simulink model "example_of_convert_unit"  (R2021a)
settings: Solver=VariableStepAuto  StartTime=0.0  StopTime=10.0  RelTol=1e-3
settings Model: Creator=YasserNet  LastModifiedBy=YasserNet

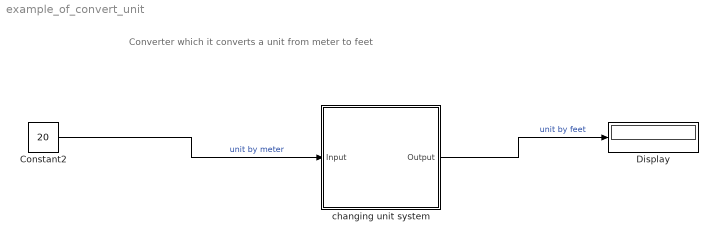
== system example_of_convert_unit ==
  note: Converter which it converts a unit from meter to feet
  Constant2 : Constant  Value=20
  Display : Display
  "changing unit system " : Subsystem
  wires:
  "changing unit system "/1(Output) -> Display/1  "unit by feet"
  Constant2/1 -> "changing unit system "/1(Input)  "unit by meter"

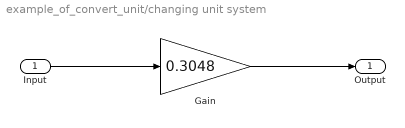
== system example_of_convert_unit/changing unit system  ==
  Input : Inport
  Gain : Gain  Gain=0.3048
  Output : Outport
  wires:
  Input/1 -> Gain/1
  Gain/1 -> Output/1
